simulink library "nist_library"  (R2012b)
settings: Solver=VariableStepDiscrete  StartTime=0  StopTime=1000  RelTol=1e-3
undefined symbols (not defined in the file or in its folder): A, B, C, D, sfp, xlipgetpartsetting
libraries: xbsIndex_r4 x385, xps_library x44, nist_library x4, casper_library_misc x4, casper_library_delays x1
(part 10 of 11)

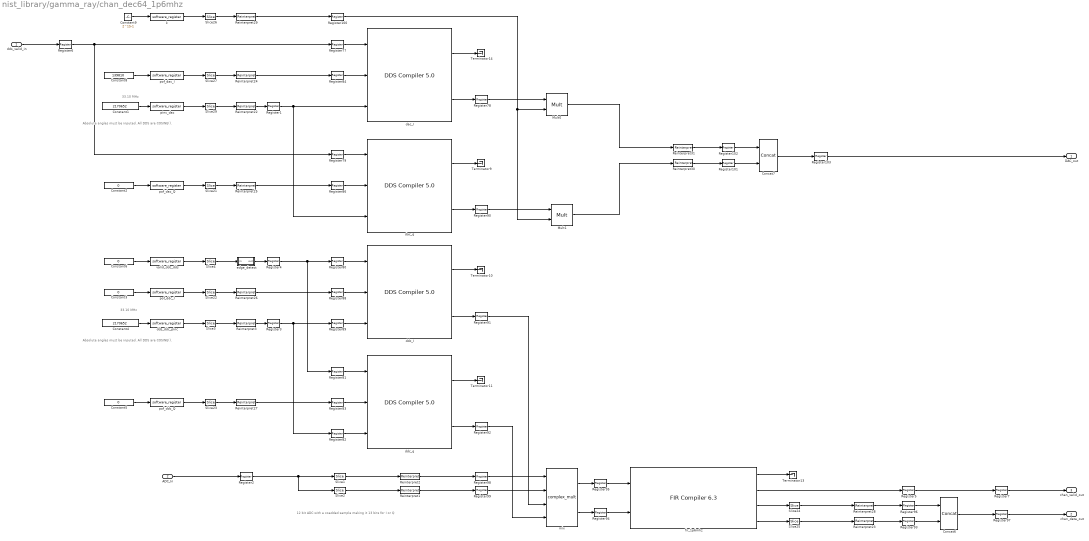
== system nist_library/gamma_ray/chan_dec64_1p6mhz ==
  note: 12 bit ADC with a coadded sample making it
      | 13 bits for I or Q
  note: Absolute angles must be inputed.
      | All DDS are COSINE().
  note: 33.10 MHz
  note: Absolute angles must be inputed.
      | All DDS are COSINE().
  note: 33.10 MHz
  dds_valid_in : Inport
  ADC_In : Inport  Port=2
  Concat6 : xbsIndex_r4/Concat  num_inputs=2  dbl_ovrd=off  block_type=concat
  Concat7 : xbsIndex_r4/Concat  num_inputs=2  dbl_ovrd=off  block_type=concat
  Constant1 : Constant  Value=2170652
  Constant{2..3,5..6} (4 alike) : Constant  Value=0
  Constant4 : Constant  Value=2170652
  Constant8 : Constant  Value=139810
  Constant9 : Constant  Value=2^15-1
  Mult0 : xbsIndex_r4/Mult  precision=User Defined  arith_type="Signed  (2's comp)"  n_bits=13  bin_pt=12  quantization=Truncate  overflow=Wrap  en=off  latency=4  dbl_ovrd=off  use_behavioral_HDL=off  opt=Area  use_embedded=off  optimum_pipeline=on  pipeline=on  use_rpm=on  placement_style=Triangular  block_type=mult
  Mult1 : xbsIndex_r4/Mult  precision=User Defined  arith_type="Signed  (2's comp)"  n_bits=13  bin_pt=12  quantization=Truncate  overflow=Wrap  en=off  latency=4  dbl_ovrd=off  use_behavioral_HDL=off  opt=Area  use_embedded=off  optimum_pipeline=on  pipeline=on  use_rpm=on  placement_style=Triangular  block_type=mult
  Register{1..7,77..84,86,88..103} (32 alike) : xbsIndex_r4/Register  init=0  rst=off  en=off  dbl_ovrd=off  block_type=register
  Reinterpret1 : xbsIndex_r4/Reinterpret  force_arith_type=on  arith_type="Signed  (2's comp)"  force_bin_pt=on  bin_pt=11  block_type=reinterpret
      settings: block_version=10.1.3
  Reinterpret2 : xbsIndex_r4/Reinterpret  force_arith_type=on  arith_type="Signed  (2's comp)"  force_bin_pt=on  bin_pt=11  block_type=reinterpret
      settings: block_version=10.1.3
  Reinterpret{3,22,24..27} (6 alike) : xbsIndex_r4/Reinterpret  force_arith_type=on  arith_type="Signed  (2's comp)"  force_bin_pt=on  bin_pt=24  block_type=reinterpret
      settings: block_version=10.1.3
  Reinterpret{23,28,30..31} (4 alike) : xbsIndex_r4/Reinterpret  force_arith_type=on  arith_type=Unsigned  force_bin_pt=on  bin_pt=0  block_type=reinterpret
      settings: block_version=10.1.3
  Reinterpret29 : xbsIndex_r4/Reinterpret  force_arith_type=on  arith_type="Signed  (2's comp)"  force_bin_pt=on  bin_pt=15  block_type=reinterpret
      settings: block_version=10.1.3
  Slice1 : xbsIndex_r4/Slice  nbits=13  boolean_output=off  mode=Lower Bit Location + Width  bit1=2  base1=Binary Point of Input  bit0=13  base0=LSB of Input  dbl_ovrd=off  block_type=slice
      settings: block_version=10.1.3
  Slice2 : xbsIndex_r4/Slice  nbits=13  boolean_output=off  mode=Lower Bit Location + Width  bit1=2  base1=Binary Point of Input  bit0=0  base0=LSB of Input  dbl_ovrd=off  block_type=slice
      settings: block_version=10.1.3
  Slice{3,21..23,27,29} (6 alike) : xbsIndex_r4/Slice  nbits=24  boolean_output=off  mode=Lower Bit Location + Width  bit1=0  base1=MSB of Input  bit0=0  base0=LSB of Input  dbl_ovrd=off  block_type=slice
      settings: block_version=10.1.3
  Slice24 : xbsIndex_r4/Slice  nbits=32  boolean_output=off  mode=Two Bit Locations  bit1=2  base1=Binary Point of Input  bit0=-18  base0=Binary Point of Input  dbl_ovrd=off  block_type=slice
      settings: block_version=10.1.3
  Slice25 : xbsIndex_r4/Slice  nbits=32  boolean_output=off  mode=Two Bit Locations  bit1=2  base1=Binary Point of Input  bit0=-18  base0=Binary Point of Input  dbl_ovrd=off  block_type=slice
      settings: block_version=10.1.3
  Slice26 : xbsIndex_r4/Slice  nbits=16  boolean_output=off  mode=Lower Bit Location + Width  bit1=0  base1=MSB of Input  bit0=0  base0=LSB of Input  dbl_ovrd=off  block_type=slice
      settings: block_version=10.1.3
  Slice4 : xbsIndex_r4/Slice  nbits=24  boolean_output=on  mode=Lower Bit Location + Width  bit1=0  base1=MSB of Input  bit0=0  base0=LSB of Input  dbl_ovrd=off  block_type=slice
      settings: block_version=10.1.3
  Terminator{9..11,13..14} (5 alike) : Terminator
  dac_I : xbsIndex_r4/DDS Compiler 5.0   partspresent=Phase_Generator_and_SIN_COS_LUT  dds_clock_rate=256  channels=1  parameter_entry=Hardware_Parameters  spurious_free_dynamic_range=36  frequency_resolution=0.4  noise_shaping=None  phase_width=24  output_width=13  output_selection=Cosine  negative_sine=off  negative_cosine=off  amplitude_mode=Full_Range  memory_type=Block_ROM  optimization_goal=Speed  dsp48_use=Minimal  latency_configuration=Auto  latency=8  has_phase_out=off  has_aclken=off  has_aresetn=off  explicit_period=off  period=1  data_has_tlast=Not_Required  has_tready=off  s_phase_has_tuser=Not_Required  m_data_has_tuser=Not_Required  m_phase_has_tuser=Not_Required  s_phase_tuser_width=1  s_config_sync_mode=On_Vector  phase_increment=Programmable  output_frequency1=0  output_frequency2=0  output_frequency3=0  output_frequency4=0  output_frequency5=0  output_frequency6=0  output_frequency7=0  output_frequency8=0  output_frequency9=0  output_frequency10=0  output_frequency11=0  output_frequency12=0  output_frequency13=0  output_frequency14=0  output_frequency15=0  output_frequency16=0  pinc1='1101000110110'  pinc2='0'  pinc3='0'  pinc4='0'  pinc5='0'  pinc6='0'  pinc7='0'  pinc8='0'  pinc9='0'  pinc10='0'  pinc11='0'  pinc12='0'  pinc13='0'  pinc14='0'  pinc15='0'  pinc16='0'  phase_offset=Programmable  phase_offset_angles1=0  phase_offset_angles2=0  phase_offset_angles3=0  phase_offset_angles4=0  phase_offset_angles5=0  phase_offset_angles6=0  phase_offset_angles7=0  phase_offset_angles8=0  phase_offset_angles9=0  phase_offset_angles10=0  phase_offset_angles11=0  phase_offset_angles12=0  phase_offset_angles13=0  phase_offset_angles14=0  phase_offset_angles15=0  phase_offset_angles16=0  poff1='0'  poff2='0'  poff3='0'  poff4='0'  poff5='0'  poff6='0'  poff7='0'  poff8='0'  poff9='0'  poff10='0'  poff11='0'  poff12='0'  poff13='0'  poff14='0'  poff15='0'  poff16='0'  trim_axipin_name=on  por_mode=false  gui_behaviour=Sysgen  ip_name=DDS Compiler  ip_version=5.0  dsptool_ready=true  wrapper_available=true  port_translation_map={ 'aclken' => 'en', 'aresetn' => 'rst' }  ipcore_xco_need_fpga_part=true  ipcore_fpga_part=xlipgetpartsetting(gcb, {'virtex6', 'xc6vlx75t', '-3', 'ff784'})  ipcore_usecache=true  ipcore_useipmodelcache=true  ipcore_verbose=false  block_type=dds_compiler_v5_0
  dac_q : xbsIndex_r4/DDS Compiler 5.0   partspresent=Phase_Generator_and_SIN_COS_LUT  dds_clock_rate=256  channels=1  parameter_entry=Hardware_Parameters  spurious_free_dynamic_range=36  frequency_resolution=0.4  noise_shaping=None  phase_width=24  output_width=13  output_selection=Sine  negative_sine=off  negative_cosine=off  amplitude_mode=Full_Range  memory_type=Block_ROM  optimization_goal=Speed  dsp48_use=Minimal  latency_configuration=Auto  latency=8  has_phase_out=off  has_aclken=off  has_aresetn=off  explicit_period=off  period=1  data_has_tlast=Not_Required  has_tready=off  s_phase_has_tuser=Not_Required  m_data_has_tuser=Not_Required  m_phase_has_tuser=Not_Required  s_phase_tuser_width=1  s_config_sync_mode=On_Vector  phase_increment=Programmable  output_frequency1=0  output_frequency2=0  output_frequency3=0  output_frequency4=0  output_frequency5=0  output_frequency6=0  output_frequency7=0  output_frequency8=0  output_frequency9=0  output_frequency10=0  output_frequency11=0  output_frequency12=0  output_frequency13=0  output_frequency14=0  output_frequency15=0  output_frequency16=0  pinc1='1101000110110'  pinc2='0'  pinc3='0'  pinc4='0'  pinc5='0'  pinc6='0'  pinc7='0'  pinc8='0'  pinc9='0'  pinc10='0'  pinc11='0'  pinc12='0'  pinc13='0'  pinc14='0'  pinc15='0'  pinc16='0'  phase_offset=Programmable  phase_offset_angles1=0  phase_offset_angles2=0  phase_offset_angles3=0  phase_offset_angles4=0  phase_offset_angles5=0  phase_offset_angles6=0  phase_offset_angles7=0  phase_offset_angles8=0  phase_offset_angles9=0  phase_offset_angles10=0  phase_offset_angles11=0  phase_offset_angles12=0  phase_offset_angles13=0  phase_offset_angles14=0  phase_offset_angles15=0  phase_offset_angles16=0  poff1='0'  poff2='0'  poff3='0'  poff4='0'  poff5='0'  poff6='0'  poff7='0'  poff8='0'  poff9='0'  poff10='0'  poff11='0'  poff12='0'  poff13='0'  poff14='0'  poff15='0'  poff16='0'  trim_axipin_name=on  por_mode=false  gui_behaviour=Sysgen  ip_name=DDS Compiler  ip_version=5.0  dsptool_ready=true  wrapper_available=true  port_translation_map={ 'aclken' => 'en', 'aresetn' => 'rst' }  ipcore_xco_need_fpga_part=true  ipcore_fpga_part=xlipgetpartsetting(gcb, {'virtex6', 'xc6vlx75t', '-3', 'ff784'})  ipcore_usecache=true  ipcore_useipmodelcache=true  ipcore_verbose=false  block_type=dds_compiler_v5_0
  ddc_I : xbsIndex_r4/DDS Compiler 5.0   partspresent=Phase_Generator_and_SIN_COS_LUT  dds_clock_rate=256  channels=1  parameter_entry=Hardware_Parameters  spurious_free_dynamic_range=36  frequency_resolution=0.4  noise_shaping=None  phase_width=24  output_width=13  output_selection=Cosine  negative_sine=off  negative_cosine=off  amplitude_mode=Full_Range  memory_type=Block_ROM  optimization_goal=Speed  dsp48_use=Minimal  latency_configuration=Auto  latency=8  has_phase_out=off  has_aclken=off  has_aresetn=off  explicit_period=off  period=1  data_has_tlast=Not_Required  has_tready=off  s_phase_has_tuser=Not_Required  m_data_has_tuser=Not_Required  m_phase_has_tuser=Not_Required  s_phase_tuser_width=1  s_config_sync_mode=On_Vector  phase_increment=Programmable  output_frequency1=0  output_frequency2=0  output_frequency3=0  output_frequency4=0  output_frequency5=0  output_frequency6=0  output_frequency7=0  output_frequency8=0  output_frequency9=0  output_frequency10=0  output_frequency11=0  output_frequency12=0  output_frequency13=0  output_frequency14=0  output_frequency15=0  output_frequency16=0  pinc1='1101000110110'  pinc2='0'  pinc3='0'  pinc4='0'  pinc5='0'  pinc6='0'  pinc7='0'  pinc8='0'  pinc9='0'  pinc10='0'  pinc11='0'  pinc12='0'  pinc13='0'  pinc14='0'  pinc15='0'  pinc16='0'  phase_offset=Programmable  phase_offset_angles1=0  phase_offset_angles2=0  phase_offset_angles3=0  phase_offset_angles4=0  phase_offset_angles5=0  phase_offset_angles6=0  phase_offset_angles7=0  phase_offset_angles8=0  phase_offset_angles9=0  phase_offset_angles10=0  phase_offset_angles11=0  phase_offset_angles12=0  phase_offset_angles13=0  phase_offset_angles14=0  phase_offset_angles15=0  phase_offset_angles16=0  poff1='0'  poff2='0'  poff3='0'  poff4='0'  poff5='0'  poff6='0'  poff7='0'  poff8='0'  poff9='0'  poff10='0'  poff11='0'  poff12='0'  poff13='0'  poff14='0'  poff15='0'  poff16='0'  trim_axipin_name=on  por_mode=false  gui_behaviour=Sysgen  ip_name=DDS Compiler  ip_version=5.0  dsptool_ready=true  wrapper_available=true  port_translation_map={ 'aclken' => 'en', 'aresetn' => 'rst' }  ipcore_xco_need_fpga_part=true  ipcore_fpga_part=xlipgetpartsetting(gcb, {'virtex6', 'xc6vlx75t', '-3', 'ff784'})  ipcore_usecache=true  ipcore_useipmodelcache=true  ipcore_verbose=false  block_type=dds_compiler_v5_0
  ddc_q : xbsIndex_r4/DDS Compiler 5.0   partspresent=Phase_Generator_and_SIN_COS_LUT  dds_clock_rate=256  channels=1  parameter_entry=Hardware_Parameters  spurious_free_dynamic_range=36  frequency_resolution=0.4  noise_shaping=None  phase_width=24  output_width=13  output_selection=Sine  negative_sine=off  negative_cosine=off  amplitude_mode=Full_Range  memory_type=Block_ROM  optimization_goal=Speed  dsp48_use=Minimal  latency_configuration=Auto  latency=8  has_phase_out=off  has_aclken=off  has_aresetn=off  explicit_period=off  period=1  data_has_tlast=Not_Required  has_tready=off  s_phase_has_tuser=Not_Required  m_data_has_tuser=Not_Required  m_phase_has_tuser=Not_Required  s_phase_tuser_width=1  s_config_sync_mode=On_Vector  phase_increment=Programmable  output_frequency1=0  output_frequency2=0  output_frequency3=0  output_frequency4=0  output_frequency5=0  output_frequency6=0  output_frequency7=0  output_frequency8=0  output_frequency9=0  output_frequency10=0  output_frequency11=0  output_frequency12=0  output_frequency13=0  output_frequency14=0  output_frequency15=0  output_frequency16=0  pinc1='1101000110110'  pinc2='0'  pinc3='0'  pinc4='0'  pinc5='0'  pinc6='0'  pinc7='0'  pinc8='0'  pinc9='0'  pinc10='0'  pinc11='0'  pinc12='0'  pinc13='0'  pinc14='0'  pinc15='0'  pinc16='0'  phase_offset=Programmable  phase_offset_angles1=0  phase_offset_angles2=0  phase_offset_angles3=0  phase_offset_angles4=0  phase_offset_angles5=0  phase_offset_angles6=0  phase_offset_angles7=0  phase_offset_angles8=0  phase_offset_angles9=0  phase_offset_angles10=0  phase_offset_angles11=0  phase_offset_angles12=0  phase_offset_angles13=0  phase_offset_angles14=0  phase_offset_angles15=0  phase_offset_angles16=0  poff1='0'  poff2='0'  poff3='0'  poff4='0'  poff5='0'  poff6='0'  poff7='0'  poff8='0'  poff9='0'  poff10='0'  poff11='0'  poff12='0'  poff13='0'  poff14='0'  poff15='0'  poff16='0'  trim_axipin_name=on  por_mode=false  gui_behaviour=Sysgen  ip_name=DDS Compiler  ip_version=5.0  dsptool_ready=true  wrapper_available=true  port_translation_map={ 'aclken' => 'en', 'aresetn' => 'rst' }  ipcore_xco_need_fpga_part=true  ipcore_fpga_part=xlipgetpartsetting(gcb, {'virtex6', 'xc6vlx75t', '-3', 'ff784'})  ipcore_usecache=true  ipcore_useipmodelcache=true  ipcore_verbose=false  block_type=dds_compiler_v5_0
  dds_ddc_pinc : xps_library/software_register  Tag=xps:sw_reg  mode=one value  io_dir=From Processor  io_delay=0  sample_period=1  names=reg  bitwidths=32  arith_types=0  bin_pts=0  sim_port=on  show_format=off
      settings: AttributesFormatString=1input
  edge_detect : Subsystem  AncestorBlock=casper_library_misc/edge_detect  mask(edge_detect){edge=Rising, polarity=Active High, x_in=[0 0.08 0.08 0.16 0.16 0.24 0.24 0.32 0.32 0.4], y_in=[-1 -1  1  1  1  1  1  1  1  1], x_out=[0.6 0.68 0.68 0.76 0.76 0.84 0.84 0.92 0.92 1], y_out=[-1 -1  1  1 -1 -1 -1 -1 -1 -1]}
      mask prompts: edge "Edge Type"; polarity "Output Polarity"; x_in "Input X Positions"; y_in "Input Y Positions"; x_out "Output X Positions"; y_out "Output Y Positions"
      mask help: Output is active for one-cycle after each edge of the specified type (i.e. rising, falling or both).
      mask init: same as nist_library/ac_bias/chan/edge_detect
      settings: AttributesFormatString=|
      | rising edges
      | active high
      mask Help: Output is active for one-cycle after each edge of the specified type (i.e. rising, falling, or both).  Latency is zero.
      mask TypeOptions edge: Rising | Falling | Both
      mask TypeOptions polarity: Active High | Active Low
      mask Display:
      | plot(x_in_num,0.5+y_in_num*0.2);
      | plot(x_out_num,0.5+y_out_num*0.2);
  fir_1p6mhz : xbsIndex_r4/FIR Compiler 6.3   coefficientvector=[0.0000019011525033,0.0000056876219913,0.0000088716128612,0.0000105285054490,0.0000112331441259,0.0000116537535111,0.0000121086815606,0.0000127062873046,0.0000134578037054,0.0000143550536492,0.0000153759219387,0.0000165069807050,0.0000177365099892,0.0000190613170757,0.0000204760588457,0.0000219808614658,0.0000235730524483,0.0000252526736666,0.0000270200365132,0.0000288801775797,0.0000308341560091,0.0000328835652662,0.0000350293217979,0.0000372743393354,0.0000396202301464,0.0000420713537247,0.0000446303739244,0.0000473006801030,0.0000500846205746,0.0000529843011946,0.0000560008044492,0.0000591383043264,0.0000624001958305,0.0000657909745546,0.0000693149655579,0.0000729755963644,0.0000767749731386,0.0000807164751480,0.0000848020183276,0.0000890348640845,0.0000934181948278,0.0000979553981420,0.0001026500574079,0.0001075058965388,0.0001125258935049,0.0001177141220482,0.0001230738041911,0.0001286088454194,0.0001343221676165,0.0001402168417012,0.0001462962205654,0.0001525635380519,0.0001590222210653,0.0001656762117708,0.0001725285293473,0.0001795829499288,0.0001868423169023,0.0001943098632186,0.0002019887062608,0.0002098823204012,0.0002179941478544,0.0002263275823252,0.0002348858565204,0.0002436717886129,0.0002526881568203,0.0002619382052226,0.0002714245815855,0.0002811507423384,0.0002911196011447,0.0003013344379480,0.0003117981572709,0.0003225137065665,0.0003334837843978,0.0003447111997165,0.0003561986265885,0.0003679485114254,0.0003799633228478,0.0003922454275732,0.0004047972499312,0.0004176213265112,0.0004307199750362,0.0004440956900758,0.0004577503480079,0.0004716861238658,0.0004859047113762,0.0005004079726070,0.0005151975978342,0.0005302755006850,0.0005456432072327,0.0005613024336877,0.0005772543894405,0.0005935003060549,0.0006100414488252,0.0006268788806523,0.0006440136970092,0.0006614468707951,0.0006791792199717,0.0006972114330779,0.0007155440150936,0.0007341773779088,0.0007531117666291,0.0007723474115159,0.0007918843489643,0.0008117225325360,0.0008318617576452,0.0008523018252725,0.0008730423006654,0.0008940828817549,0.0009154227821344,0.0009370612914688,0.0009589972459099,0.0009812295942941,0.0010037569518702,0.0010265779915594,0.0010496912108847,0.0010730951039130,0.0010967878087028,0.0011207675003003,0.0011450318860620,0.0011695787995345,0.0011944057911537,0.0012195103635321,0.0012448898147327,0.0012705413569648,0.0012964619391775,0.0013226484391489,0.0013490975727786,0.0013758058780469,0.0014027697964972,0.0014299856403171,0.0014574495015892,0.0014851574058773,0.0015131051294534,0.0015412884060349,0.0015697027987165,0.0015983436869004,0.0016272062935310,0.0016562855988542,0.0016855765416188,0.0017150738655039,0.0017447722386838,0.0017746662255090,0.0018047502445680,0.0018350185631017,0.0018654652539320,0.0018960842434900,0.0019268692651770,0.0019578140116174,0.0019889120122188,0.0020201567134556,0.0020515413937462,0.0020830592380900,0.0021147032494305,0.0021464663868889,0.0021783414401616,0.0022103210597356,0.0022423978324420,0.0022745641940544,0.0023068124318291,0.0023391348084616,0.0023715233689647,0.0024039702204384,0.0024364672341703,0.0024690062752231,0.0025015789926230,0.0025341770485584,0.0025667919451159,0.0025994152113847,0.0026320382185188,0.0026646523522306,0.0026972488120066,0.0027298187899910,0.0027623533239569,0.0027948434403345,0.0028272800542585,0.0028596541468211,0.0028919565693448,0.0029241781950509,0.0029563097841795,0.0029883421071597,0.0030202658407632,0.0030520717295471,0.0030837503376857,0.0031152923584850,0.0031466883355585,0.0031779289147561,0.0032090046318295,0.0032399061370104,0.0032706239877962,0.0033011488459664,0.0033314712893272,0.0033615819555686,0.0033914714144453,0.0034211303633995,0.0034505494290623,0.0034797194024499,0.0035086309882751,0.0035372750121209,0.0035656422670832,0.0035937236431558,0.0036215100360043,0.0036489924398562,0.0036761618873479,0.0037030095592243,0.0037295266062674,0.0037557043424330,0.0037815340620543,0.0038070072264042,0.0038321153197985,0.0038568499906846 ...(+5757 chars)]  coefficient_sets=1  coefficient_reload=off  filter_type=Decimation  rate_change_type=Integer  interpolation_rate=1  decimation_rate=64  zero_pack_factor=1  channel_sequence=Basic  number_channels=1  pattern_list='P4-0,P4-1,P4-2,P4-3,P4-4'  number_paths=2  ratespecification=Maximum_Possible  sampleperiod=1  hardwareoversamplingrate=1  coefficient_sign=Unsigned  quantization=Maximize_Dynamic_Range  coefficient_width=14  bestprecision=on  coefficient_fractional_bits=21  coefficient_structure=Inferred  output_rounding_mode=Full_Precision  output_width=38  filter_architecture=Systolic_Multiply_Accumulate  optimization_goal=Area  data_buffer_type=Automatic  coefficient_buffer_type=Automatic  input_buffer_type=Not_Applicable  output_buffer_type=Not_Applicable  preference_for_other_storage=Automatic  multi_column_support=Automatic  columnconfig='5'  inter_column_pipe_length=4  data_has_tlast=Not_Required  m_data_has_tready=off  s_data_has_fifo=off  s_data_has_tuser=Not_Required  m_data_has_tuser=Not_Required  s_config_sync_mode=On_Vector  s_config_method=Single  num_reload_slots=1  has_aclken=off  has_aresetn=off  infoeditControl=ARESETn must be asserted for a minimum of 2 cycles  trim_axipin_name=on  passband_min=0.0  passband_max=0.5  stopband_min=0.5  stopband_max=1.0  filter_selection=1  gui_behaviour=Sysgen_GUI  data_sign=Signed  data_width=16  data_fractional_bits=0  data_tuser_width=1  wrapper_available=true  ip_wrap_arbitrary_binary_point=true  ip_name=FIR Compiler  ip_version=6.3  dsptool_ready=true  ipcore_usecache=true  ipcore_useipmodelcache=true  ipcore_xco_need_fpga_part=true  port_translation_map={ 'aclken' => 'en', 'aresetn' => 'rst' }  run_core_at_system_period=true  ipcore_fpga_part=xlipgetpartsetting(gcb, {'virtex6', 'xc6vlx75t', '-3', 'ff784'})  block_type=fir_compiler_v6_3
      settings: infoedit=Maximum Possible : Maximizes oversampling rate. Abstracted input handshake (no s_data_tvalid) and automatic rate propagation.<br>Hardware Oversampling Rate : Specifies oversampling rate relative to the input sample period. Abstracted input handshake (no s_data_tvalid) and automatic rate propagation.<br>Sample Period : Specifies absolute oversampling rate. No input handshake abstraction (exposes s_data_tvalid) and no rate propagation.
  k : xps_library/software_register  Tag=xps:sw_reg  mode=one value  io_dir=From Processor  io_delay=0  sample_period=1  names=reg  bitwidths=32  arith_types=0  bin_pts=0  sim_port=on  show_format=off
      settings: AttributesFormatString=1input
  mix : nist_library/utility/complex_mult
  pinc_dac : xps_library/software_register  Tag=xps:sw_reg  mode=one value  io_dir=From Processor  io_delay=0  sample_period=1  names=reg  bitwidths=32  arith_types=0  bin_pts=0  sim_port=on  show_format=off
      settings: AttributesFormatString=1input
  pof_dac_I : xps_library/software_register  Tag=xps:sw_reg  mode=one value  io_dir=From Processor  io_delay=0  sample_period=1  names=reg  bitwidths=32  arith_types=0  bin_pts=0  sim_port=on  show_format=off
      settings: AttributesFormatString=1input
  pof_dac_Q : xps_library/software_register  Tag=xps:sw_reg  mode=one value  io_dir=From Processor  io_delay=0  sample_period=1  names=reg  bitwidths=32  arith_types=0  bin_pts=0  sim_port=on  show_format=off
      settings: AttributesFormatString=1input
  pof_ddc_I : xps_library/software_register  Tag=xps:sw_reg  mode=one value  io_dir=From Processor  io_delay=0  sample_period=1  names=reg  bitwidths=32  arith_types=0  bin_pts=0  sim_port=on  show_format=off
      settings: AttributesFormatString=1input
  pof_ddc_Q : xps_library/software_register  Tag=xps:sw_reg  mode=one value  io_dir=From Processor  io_delay=0  sample_period=1  names=reg  bitwidths=32  arith_types=0  bin_pts=0  sim_port=on  show_format=off
      settings: AttributesFormatString=1input
  valid_ddc_dds : xps_library/software_register  Tag=xps:sw_reg  mode=one value  io_dir=From Processor  io_delay=0  sample_period=1  names=reg  bitwidths=32  arith_types=0  bin_pts=0  sim_port=on  show_format=off
      settings: AttributesFormatString=1input
  DAC_out : Outport
  chan_data_out : Outport  Port=2
  chan_valid_out : Outport  Port=3
  wires:
  Reinterpret29/1 -> Register100/1
  Register101/1 -> Concat7/2
  Register102/1 -> Concat7/1
  Mult0/1 -> Reinterpret31/1
  Constant9/1 -> k/1
  Slice26/1 -> Reinterpret29/1
  k/1 -> Slice26/1
  Register78/1 -> Mult0/1
  ddc_q/2 -> Register92/1
  Constant3/1 -> pof_ddc_I/1
  fir_1p6mhz/4 -> Slice25/1
  fir_1p6mhz/1 -> Terminator13/1
  Slice24/1 -> Reinterpret28/1
  Slice25/1 -> Reinterpret23/1
  dac_q/2 -> Register90/1
  Mult1/1 -> Reinterpret30/1
  ddc_I/2 -> Register91/1
  Register82/1 -> ddc_q/3
  Register84/1 -> dac_I/2
  dac_I/2 -> Register78/1
  ddc_I/1 -> Terminator10/1
  ddc_q/1 -> Terminator11/1
  Reinterpret24/1 -> Register84/1
  Slice22/1 -> Reinterpret26/1
  Register103/1 -> DAC_out/1
  Register83/1 -> ddc_q/2
  Register1/1 -> dac_I/3, dac_q/3
  Register81/1 -> ddc_q/1
  Reinterpret26/1 -> Register88/1
  Slice21/1 -> Reinterpret25/1
  dac_q/1 -> Terminator9/1
  Register99/1 -> mix/2
  Register97/1 -> chan_data_out/1
  mix/2 -> Register94/1
  mix/1 -> Register95/1
  Concat6/1 -> Register97/1
  Reinterpret23/1 -> Register93/1
  Reinterpret28/1 -> Register96/1
  Register95/1 -> fir_1p6mhz/1
  Register94/1 -> fir_1p6mhz/2
  fir_1p6mhz/2 -> Register5/1
  Register93/1 -> Concat6/2
  Register96/1 -> Concat6/1
  fir_1p6mhz/3 -> Slice24/1
  Register90/1 -> Mult1/1
  Reinterpret31/1 -> Register102/1
  Reinterpret30/1 -> Register101/1
  Register86/1 -> dac_q/2
  Register98/1 -> mix/1
  Register89/1 -> ddc_I/3
  Reinterpret27/1 -> Register83/1
  Concat7/1 -> Register103/1
  pof_ddc_I/1 -> Slice22/1
  Register88/1 -> ddc_I/2
  Register80/1 -> ddc_I/1
  Register100/1 -> Mult1/2, Mult0/2
  Reinterpret25/1 -> Register86/1
  Reinterpret22/1 -> Register1/1
  Slice23/1 -> Reinterpret27/1
  Constant5/1 -> pof_ddc_Q/1
  pof_ddc_Q/1 -> Slice23/1
  Constant1/1 -> pinc_dac/1
  dds_valid_in/1 -> Register6/1
  dac_I/1 -> Terminator14/1
  Slice27/1 -> Reinterpret24/1
  Slice29/1 -> Reinterpret22/1
  Register77/1 -> dac_I/1
  Constant8/1 -> pof_dac_I/1
  pof_dac_I/1 -> Slice27/1
  pinc_dac/1 -> Slice29/1
  Register79/1 -> dac_q/1
  Constant2/1 -> pof_dac_Q/1
  pof_dac_Q/1 -> Slice21/1
  Slice1/1 -> Reinterpret2/1
  Slice2/1 -> Reinterpret1/1
  ADC_In/1 -> Register2/1
  Register2/1 -> Slice2/1, Slice1/1
  Reinterpret2/1 -> Register98/1
  Reinterpret1/1 -> Register99/1
  Register6/1 -> Register79/1, Register77/1
  Register3/1 -> Register82/1, Register89/1
  Register91/1 -> mix/3
  Register92/1 -> mix/4
  Constant4/1 -> dds_ddc_pinc/1
  dds_ddc_pinc/1 -> Slice3/1
  Constant6/1 -> valid_ddc_dds/1
  valid_ddc_dds/1 -> Slice4/1
  Slice4/1 -> edge_detect/1(in)
  Slice3/1 -> Reinterpret3/1
  Reinterpret3/1 -> Register3/1
  edge_detect/1(out) -> Register4/1
  Register4/1 -> Register81/1, Register80/1
  Register5/1 -> Register7/1
  Register7/1 -> chan_valid_out/1

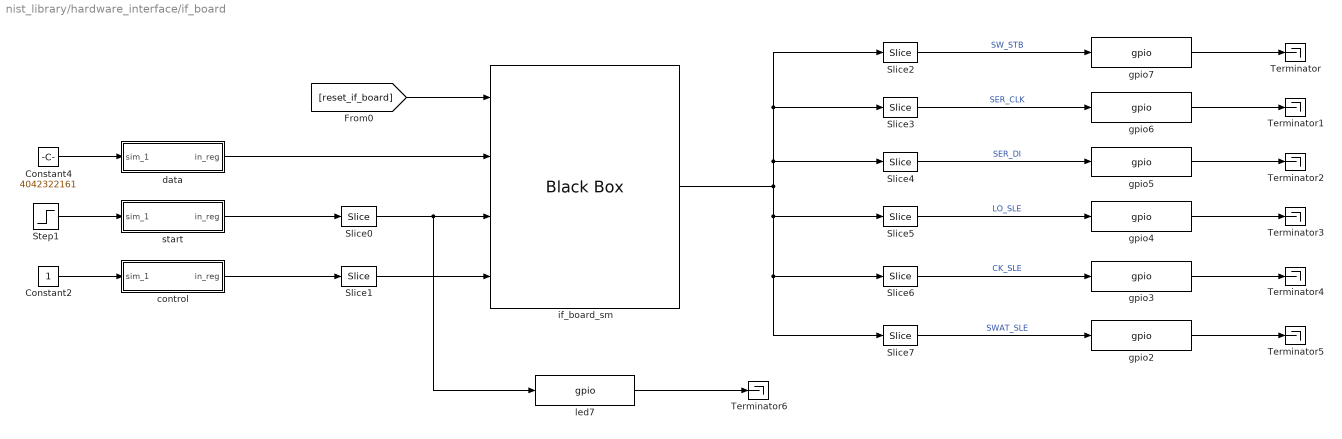
== system nist_library/hardware_interface/if_board ==
  Constant2 : Constant
  Constant4 : Constant  Value=4042322161
  Slice0 : xbsIndex_r4/Slice  nbits=1  boolean_output=on  mode=Lower Bit Location + Width  bit1=0  base1=MSB of Input  bit0=0  base0=LSB of Input  dbl_ovrd=off  block_type=slice
  Slice1 : xbsIndex_r4/Slice  nbits=4  boolean_output=off  mode=Lower Bit Location + Width  bit1=0  base1=MSB of Input  bit0=0  base0=LSB of Input  dbl_ovrd=off  block_type=slice
  Slice2 : xbsIndex_r4/Slice  nbits=4  boolean_output=on  mode=Lower Bit Location + Width  bit1=0  base1=MSB of Input  bit0=0  base0=LSB of Input  dbl_ovrd=off  block_type=slice
  Slice3 : xbsIndex_r4/Slice  nbits=4  boolean_output=on  mode=Lower Bit Location + Width  bit1=0  base1=MSB of Input  bit0=1  base0=LSB of Input  dbl_ovrd=off  block_type=slice
  Slice4 : xbsIndex_r4/Slice  nbits=4  boolean_output=on  mode=Lower Bit Location + Width  bit1=0  base1=MSB of Input  bit0=2  base0=LSB of Input  dbl_ovrd=off  block_type=slice
  Slice5 : xbsIndex_r4/Slice  nbits=4  boolean_output=on  mode=Lower Bit Location + Width  bit1=0  base1=MSB of Input  bit0=3  base0=LSB of Input  dbl_ovrd=off  block_type=slice
  Slice6 : xbsIndex_r4/Slice  nbits=4  boolean_output=on  mode=Lower Bit Location + Width  bit1=0  base1=MSB of Input  bit0=4  base0=LSB of Input  dbl_ovrd=off  block_type=slice
  Slice7 : xbsIndex_r4/Slice  nbits=4  boolean_output=on  mode=Lower Bit Location + Width  bit1=0  base1=MSB of Input  bit0=5  base0=LSB of Input  dbl_ovrd=off  block_type=slice
  Step1 : Step  Time=20  SampleTime=1
  Terminator{,1..6} (7 alike) : Terminator
  control : Subsystem  Tag=xps:sw_reg  AncestorBlock=xps_library/software register  mask(swreg){mode=one value, io_dir=From Processor, io_delay=0, sample_period=1, names=reg, bitwidths=32, arith_types=0, bin_pts=0, sim_port=on, show_format=off}
      mask prompts: io_dir "I/O direction"; io_delay "I/O delay"; sample_period "Sample period"; names "Name:"; bitwidths "Bitwidth:"; arith_types "Type (ufix=0, fix=1, bool=2):"; bin_pts "Binary pt:"; sim_port "Provide sim input/output?"; show_format "Print format string?"
      mask init:
      | swreg_init(gcb)
      settings: AttributesFormatString=1input
      mask TypeOptions mode: one value | fields of equal size | fields of arbitrary size
      mask Callback mode: swreg_cb(gcb);
      mask TypeOptions io_dir: To Processor | From Processor
      mask Callback io_dir:
      | mask_enables = get_param(gcb, 'MaskEnables');
      | mask_names = get_param(gcb, 'MaskNames');
      | if strcmp(get_param(gcb, 'io_dir'), 'To Processor'),
      |     mask_enables{ismember(mask_names, 'sample_period')} = 'off';
      | else
      |     mask_enables{ismember(mask_names, 'sample_period')} = 'on';
      | end
      | set_param(gcb, 'MaskEnables', mask_enables);
      mask Callback bitwidths: swreg_maskcheck(gcb);
      mask Callback arith_types: [numios, ~, ~, ~, current_types] = swreg_maskcheck(gcb);
      mask Callback bin_pts: swreg_maskcheck(gcb);
  data : Subsystem  Tag=xps:sw_reg  AncestorBlock=xps_library/software register  mask(swreg){mode=one value, io_dir=From Processor, io_delay=0, sample_period=1, names=reg, bitwidths=32, arith_types=0, bin_pts=0, sim_port=on, show_format=off}
      mask prompts: io_dir "I/O direction"; io_delay "I/O delay"; sample_period "Sample period"; names "Name:"; bitwidths "Bitwidth:"; arith_types "Type (ufix=0, fix=1, bool=2):"; bin_pts "Binary pt:"; sim_port "Provide sim input/output?"; show_format "Print format string?"
      mask init:
      | swreg_init(gcb)
      settings: AttributesFormatString=1input
      mask TypeOptions mode: one value | fields of equal size | fields of arbitrary size
      mask Callback mode: swreg_cb(gcb);
      mask TypeOptions io_dir: To Processor | From Processor
      mask Callback io_dir:
      | mask_enables = get_param(gcb, 'MaskEnables');
      | mask_names = get_param(gcb, 'MaskNames');
      | if strcmp(get_param(gcb, 'io_dir'), 'To Processor'),
      |     mask_enables{ismember(mask_names, 'sample_period')} = 'off';
      | else
      |     mask_enables{ismember(mask_names, 'sample_period')} = 'on';
      | end
      | set_param(gcb, 'MaskEnables', mask_enables);
      mask Callback bitwidths: swreg_maskcheck(gcb);
      mask Callback arith_types: [numios, ~, ~, ~, current_types] = swreg_maskcheck(gcb);
      mask Callback bin_pts: swreg_maskcheck(gcb);
  gpio2 : xps_library/gpio  Tag=xps:gpio  io_group=ROACH2:gpio  io_dir=out  arith_type=Unsigned  bitwidth=1  bin_pt=0  bit_index=2  sample_period=1  use_single_ended=off  use_ddr=off  reg_iob=on  reg_clk_phase=0  termination=None
  gpio3 : xps_library/gpio  Tag=xps:gpio  io_group=ROACH2:gpio  io_dir=out  arith_type=Unsigned  bitwidth=1  bin_pt=0  bit_index=3  sample_period=1  use_single_ended=off  use_ddr=off  reg_iob=on  reg_clk_phase=0  termination=None
  gpio4 : xps_library/gpio  Tag=xps:gpio  io_group=ROACH2:gpio  io_dir=out  arith_type=Unsigned  bitwidth=1  bin_pt=0  bit_index=4  sample_period=1  use_single_ended=off  use_ddr=off  reg_iob=on  reg_clk_phase=0  termination=None
  gpio5 : xps_library/gpio  Tag=xps:gpio  io_group=ROACH2:gpio  io_dir=out  arith_type=Unsigned  bitwidth=1  bin_pt=0  bit_index=5  sample_period=1  use_single_ended=off  use_ddr=off  reg_iob=on  reg_clk_phase=0  termination=None
  gpio6 : xps_library/gpio  Tag=xps:gpio  io_group=ROACH2:gpio  io_dir=out  arith_type=Unsigned  bitwidth=1  bin_pt=0  bit_index=6  sample_period=1  use_single_ended=off  use_ddr=off  reg_iob=on  reg_clk_phase=0  termination=None
  gpio7 : xps_library/gpio  Tag=xps:gpio  io_group=ROACH2:gpio  io_dir=out  arith_type=Unsigned  bitwidth=1  bin_pt=0  bit_index=7  sample_period=1  use_single_ended=off  use_ddr=off  reg_iob=on  reg_clk_phase=0  termination=None
  if_board_sm : xbsIndex_r4/Black Box  init_code=ROACH2_IF_SM_config  sim_method=Inactive  verbose=off  block_type=blackbox2
  led7 : xps_library/gpio  Tag=xps:gpio  io_group=ROACH2:led  io_dir=out  arith_type=Unsigned  bitwidth=1  bin_pt=0  bit_index=7  sample_period=1  use_single_ended=off  use_ddr=off  reg_iob=on  reg_clk_phase=0  termination=None
  start : Subsystem  Tag=xps:sw_reg  AncestorBlock=xps_library/software register  mask(swreg){mode=one value, io_dir=From Processor, io_delay=0, sample_period=1, names=reg, bitwidths=32, arith_types=0, bin_pts=0, sim_port=on, show_format=off}
      mask prompts: io_dir "I/O direction"; io_delay "I/O delay"; sample_period "Sample period"; names "Name:"; bitwidths "Bitwidth:"; arith_types "Type (ufix=0, fix=1, bool=2):"; bin_pts "Binary pt:"; sim_port "Provide sim input/output?"; show_format "Print format string?"
      mask init:
      | swreg_init(gcb)
      settings: AttributesFormatString=1input
      mask TypeOptions mode: one value | fields of equal size | fields of arbitrary size
      mask Callback mode: swreg_cb(gcb);
      mask TypeOptions io_dir: To Processor | From Processor
      mask Callback io_dir:
      | mask_enables = get_param(gcb, 'MaskEnables');
      | mask_names = get_param(gcb, 'MaskNames');
      | if strcmp(get_param(gcb, 'io_dir'), 'To Processor'),
      |     mask_enables{ismember(mask_names, 'sample_period')} = 'off';
      | else
      |     mask_enables{ismember(mask_names, 'sample_period')} = 'on';
      | end
      | set_param(gcb, 'MaskEnables', mask_enables);
      mask Callback bitwidths: swreg_maskcheck(gcb);
      mask Callback arith_types: [numios, ~, ~, ~, current_types] = swreg_maskcheck(gcb);
      mask Callback bin_pts: swreg_maskcheck(gcb);
  wires:
  gpio3/1 -> Terminator4/1
  start/1(in_reg) -> Slice0/1
  Slice1/1 -> if_board_sm/4
  led7/1 -> Terminator6/1
  gpio7/1 -> Terminator/1
  gpio5/1 -> Terminator2/1
  Constant2/1 -> control/1(sim_1)
  gpio4/1 -> Terminator3/1
  gpio2/1 -> Terminator5/1
  if_board_sm/1 -> Slice7/1, Slice6/1, Slice5/1, Slice2/1, Slice3/1, Slice4/1
  Constant4/1 -> data/1(sim_1)
  Step1/1 -> start/1(sim_1)
  Slice2/1 -> gpio7/1  "SW_STB"
  Slice4/1 -> gpio5/1  "SER_DI"
  Slice6/1 -> gpio3/1  "CK_SLE"
  Slice0/1 -> led7/1, if_board_sm/3
  Slice3/1 -> gpio6/1  "SER_CLK"
  control/1(in_reg) -> Slice1/1
  data/1(in_reg) -> if_board_sm/2
  Slice5/1 -> gpio4/1  "LO_SLE"
  gpio6/1 -> Terminator1/1
  Slice7/1 -> gpio2/1  "SWAT_SLE"
  [reset_if_board] -> if_board_sm/1

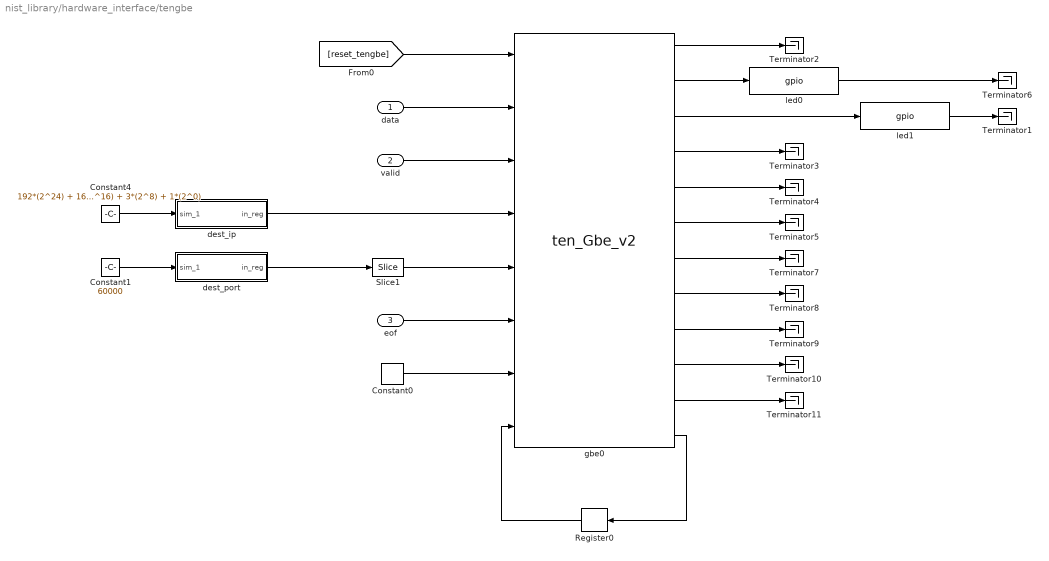
== system nist_library/hardware_interface/tengbe ==
  data : Inport
  valid : Inport  Port=2
  eof : Inport  Port=3
  Constant0 : xbsIndex_r4/Constant  const=1  gui_display_data_type=Boolean  arith_type=Boolean  n_bits=16  bin_pt=14  preci_type=Single  exp_width=8  frac_width=24  explicit_period=off  period=1  equ=P=C  opselect=C  inp2=PCIN>>17  opr=+  inp1=P  carry=CIN  dbl_ovrd=off  block_type=constant
  Constant1 : Constant  Value=60000
  Constant4 : Constant  Value=192*(2^24) + 168*(2^16) + 3*(2^8) + 1*(2^0)
  Register0 : xbsIndex_r4/Register  init=0  rst=off  en=off  dbl_ovrd=off  block_type=register
  Slice1 : xbsIndex_r4/Slice  nbits=16  boolean_output=off  mode=Lower Bit Location + Width  bit1=0  base1=MSB of Input  bit0=0  base0=LSB of Input  dbl_ovrd=off  block_type=slice
  Terminator{1..11} (11 alike) : Terminator
  dest_ip : Subsystem  Tag=xps:sw_reg  AncestorBlock=xps_library/software register  mask(swreg){mode=one value, io_dir=From Processor, io_delay=0, sample_period=1, names=reg, bitwidths=32, arith_types=0, bin_pts=0, sim_port=on, show_format=off}
      mask prompts: io_dir "I/O direction"; io_delay "I/O delay"; sample_period "Sample period"; names "Name:"; bitwidths "Bitwidth:"; arith_types "Type (ufix=0, fix=1, bool=2):"; bin_pts "Binary pt:"; sim_port "Provide sim input/output?"; show_format "Print format string?"
      mask init:
      | swreg_init(gcb)
      settings: AttributesFormatString=1input
      mask TypeOptions mode: one value | fields of equal size | fields of arbitrary size
      mask Callback mode: swreg_cb(gcb);
      mask TypeOptions io_dir: To Processor | From Processor
      mask Callback io_dir:
      | mask_enables = get_param(gcb, 'MaskEnables');
      | mask_names = get_param(gcb, 'MaskNames');
      | if strcmp(get_param(gcb, 'io_dir'), 'To Processor'),
      |     mask_enables{ismember(mask_names, 'sample_period')} = 'off';
      | else
      |     mask_enables{ismember(mask_names, 'sample_period')} = 'on';
      | end
      | set_param(gcb, 'MaskEnables', mask_enables);
      mask Callback bitwidths: swreg_maskcheck(gcb);
      mask Callback arith_types: [numios, ~, ~, ~, current_types] = swreg_maskcheck(gcb);
      mask Callback bin_pts: swreg_maskcheck(gcb);
  dest_port : Subsystem  Tag=xps:sw_reg  AncestorBlock=xps_library/software register  mask(swreg){mode=one value, io_dir=From Processor, io_delay=0, sample_period=1, names=reg, bitwidths=32, arith_types=0, bin_pts=0, sim_port=on, show_format=off}
      mask prompts: io_dir "I/O direction"; io_delay "I/O delay"; sample_period "Sample period"; names "Name:"; bitwidths "Bitwidth:"; arith_types "Type (ufix=0, fix=1, bool=2):"; bin_pts "Binary pt:"; sim_port "Provide sim input/output?"; show_format "Print format string?"
      mask init:
      | swreg_init(gcb)
      settings: AttributesFormatString=1input
      mask TypeOptions mode: one value | fields of equal size | fields of arbitrary size
      mask Callback mode: swreg_cb(gcb);
      mask TypeOptions io_dir: To Processor | From Processor
      mask Callback io_dir:
      | mask_enables = get_param(gcb, 'MaskEnables');
      | mask_names = get_param(gcb, 'MaskNames');
      | if strcmp(get_param(gcb, 'io_dir'), 'To Processor'),
      |     mask_enables{ismember(mask_names, 'sample_period')} = 'off';
      | else
      |     mask_enables{ismember(mask_names, 'sample_period')} = 'on';
      | end
      | set_param(gcb, 'MaskEnables', mask_enables);
      mask Callback bitwidths: swreg_maskcheck(gcb);
      mask Callback arith_types: [numios, ~, ~, ~, current_types] = swreg_maskcheck(gcb);
      mask Callback bin_pts: swreg_maskcheck(gcb);
  gbe0 : xps_library/ten_Gbe_v2  Tag=xps:tengbe_v2  flavour=sfp+  slot=0  port_r1=0  port_r2_cx4=0  port_r2_sfpp=0  rx_dist_ram=on  large_frames=on  show_param=off  pre_emph_r2=0.74  pre_emph=3  post_emph_r2=0.18  rxeqmix_r2=7  swing_r2=940  swing=800  fab_en=on  fab_mac=hex2dec('123456780000')  fab_ip=192*(2^24) + 168*(2^16) + 5*(2^8) + 20*(2^0)  fab_udp=10000  fab_gate=1  cpu_rx_en=on  cpu_tx_en=on  ttl=hex2dec('FF')  promisc_mode=off  debug_ctr_width=16  txctr=off  txerrctr=off  txerrctr_len=100  txofctr=off  txfullctr=off  txvldctr=off  txsnaplen=0 - no snap  rxctr=off  rxerrctr=off  rxerrctr_len=100  rxofctr=off  rxbadctr=off  rxvldctr=off  rxeofctr=off  rxsnaplen=0 - no snap
  led0 : xps_library/gpio  Tag=xps:gpio  io_group=ROACH2:led  io_dir=out  arith_type=Unsigned  bitwidth=1  bin_pt=0  bit_index=0  sample_period=1  use_single_ended=off  use_ddr=off  reg_iob=on  reg_clk_phase=0  termination=None
  led1 : xps_library/gpio  Tag=xps:gpio  io_group=ROACH2:led  io_dir=out  arith_type=Unsigned  bitwidth=1  bin_pt=0  bit_index=1  sample_period=1  use_single_ended=off  use_ddr=off  reg_iob=on  reg_clk_phase=0  termination=None
  wires:
  eof/1 -> gbe0/6
  valid/1 -> gbe0/3
  data/1 -> gbe0/2
  Constant4/1 -> dest_ip/1(sim_1)
  Constant1/1 -> dest_port/1(sim_1)
  dest_port/1(in_reg) -> Slice1/1
  [reset_tengbe] -> gbe0/1
  dest_ip/1(in_reg) -> gbe0/4
  Slice1/1 -> gbe0/5
  Constant0/1 -> gbe0/7
  gbe0/12 -> Register0/1
  Register0/1 -> gbe0/8
  led0/1 -> Terminator6/1
  led1/1 -> Terminator1/1
  gbe0/3 -> led1/1
  gbe0/2 -> led0/1
  gbe0/11 -> Terminator11/1
  gbe0/10 -> Terminator10/1
  gbe0/9 -> Terminator9/1
  gbe0/8 -> Terminator8/1
  gbe0/7 -> Terminator7/1
  gbe0/6 -> Terminator5/1
  gbe0/5 -> Terminator4/1
  gbe0/4 -> Terminator3/1
  gbe0/1 -> Terminator2/1

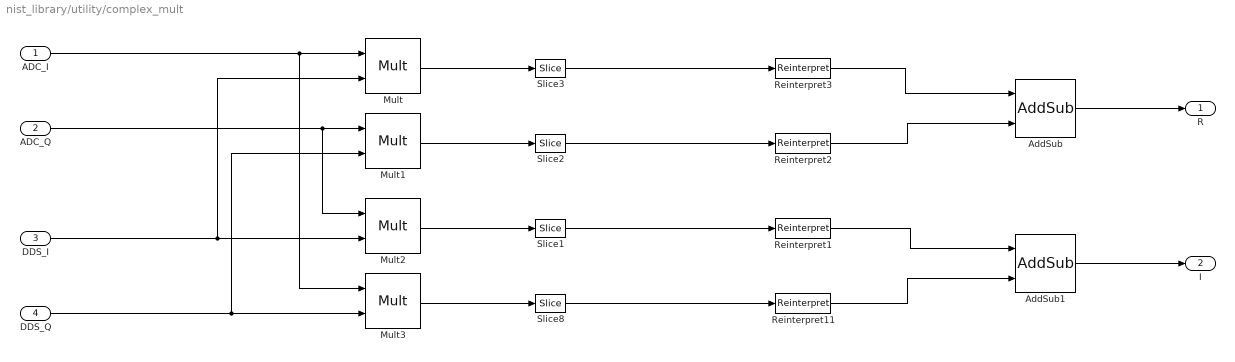
== system nist_library/utility/complex_mult ==
  ADC_I : Inport
  ADC_Q : Inport  Port=2
  DDS_I : Inport  Port=3
  DDS_Q : Inport  Port=4
  AddSub : xbsIndex_r4/AddSub  mode=Subtraction  use_carryin=off  use_carryout=off  en=off  latency=4  precision=Full  arith_type=Unsigned  n_bits=16  bin_pt=14  quantization=Truncate  overflow=Wrap  dbl_ovrd=off  use_behavioral_HDL=off  hw_selection=Fabric  pipelined=on  block_type=addsub
  AddSub1 : xbsIndex_r4/AddSub  mode=Addition  use_carryin=off  use_carryout=off  en=off  latency=4  precision=Full  arith_type=Unsigned  n_bits=16  bin_pt=14  quantization=Truncate  overflow=Wrap  dbl_ovrd=off  use_behavioral_HDL=off  hw_selection=Fabric  pipelined=on  block_type=addsub
  Mult{,1..3} (4 alike) : xbsIndex_r4/Mult  precision=Full  arith_type="Signed  (2's comp)"  n_bits=16  bin_pt=14  quantization=Truncate  overflow=Wrap  en=off  latency=4  dbl_ovrd=off  use_behavioral_HDL=off  opt=Area  use_embedded=on  optimum_pipeline=on  pipeline=on  use_rpm=on  placement_style=Triangular  block_type=mult
  Reinterpret{1..3,11} (4 alike) : xbsIndex_r4/Reinterpret  force_arith_type=on  arith_type="Signed  (2's comp)"  force_bin_pt=on  bin_pt=14  block_type=reinterpret
      settings: block_version=10.1.3
  Slice{1..3,8} (4 alike) : xbsIndex_r4/Slice  nbits=12  boolean_output=off  mode=Two Bit Locations  bit1=1  base1=Binary Point of Input  bit0=-14  base0=Binary Point of Input  dbl_ovrd=off  block_type=slice
      settings: block_version=10.1.3
  R : Outport
  I : Outport  Port=2
  wires:
  AddSub/1 -> R/1
  AddSub1/1 -> I/1
  DDS_I/1 -> Mult2/2, Mult/2
  ADC_I/1 -> Mult3/1, Mult/1
  Mult/1 -> Slice3/1
  Mult2/1 -> Slice1/1
  Mult3/1 -> Slice8/1
  DDS_Q/1 -> Mult1/2, Mult3/2
  Mult1/1 -> Slice2/1
  ADC_Q/1 -> Mult2/1, Mult1/1
  Reinterpret11/1 -> AddSub1/2
  Reinterpret1/1 -> AddSub1/1
  Reinterpret2/1 -> AddSub/2
  Reinterpret3/1 -> AddSub/1
  Slice3/1 -> Reinterpret3/1
  Slice2/1 -> Reinterpret2/1
  Slice1/1 -> Reinterpret1/1
  Slice8/1 -> Reinterpret11/1
